simulink model "questao6"  (R2023a)
settings: Solver=VariableStepAuto  StartTime=0.0  StopTime=50  RelTol=1e-3
values from neighbouring files (symbols this model uses):
  B = 0.1    [Trab1_real.m]    (also in questao5.m)
  J = 1    [Trab1_real.m]    (also in questao5.m)
  K = 1/3    (= 0.333333333333)    [Trab1_real.m]    (also in questao5.m)
  L = 0.5    [Trab1_real.m]    (also in questao5.m)
  R = 10    [Trab1_real.m]    (also in questao5.m)
settings Model: Creator=thiag  LastModifiedBy=thiag

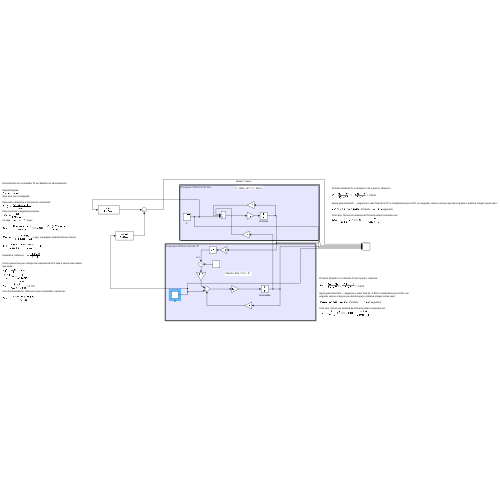
[thumbnail: Simulink's stored preview of the top-level diagram]
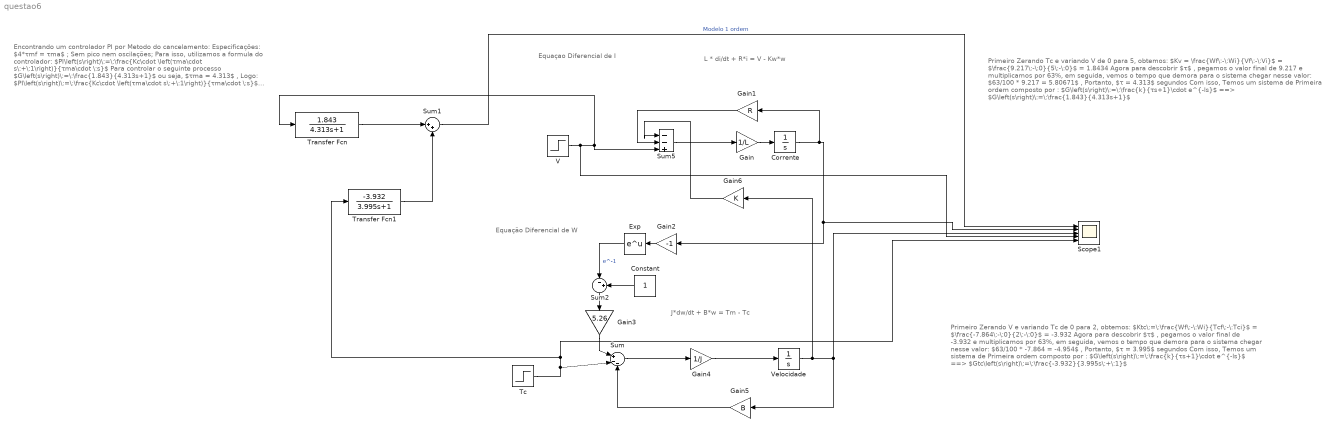
== system questao6 ==
  note: Encontrando um controlador PI por Metodo do cancelamento:
      |
      | Especificações:
      | $4*τmf = τma$ ;
      | Sem pico nem oscilações;
      |
      | Para isso, utilizamos a formula do controlador:
      | $PI\left(s\right)\:=\:\frac{Kc\cdot \left(τma\cdot s\:+\:1\right)}{τma\cdot \:s}$
      | Para controlar o seguinte processo
      | $G\left(s\right)\:=\:\frac{1.843}{4.313s+1}$
      | ou seja, $τma = 4.313$ , Logo:
      |
      | $PI\left(s\right)\:=\:\frac{Kc\cdot \left(τma\cdot s\:+\:1\right)}{τma\cdot \:s}$ ==> $PI\left(s\right)\:=\:\frac{Kc\cdot \left(4.313s+1\right)}{4.313s}$
      |
      | $Gmf\left(s\right)\:=\:\frac{C\left(s\right)\cdot G\left(s\right)}{1\:+\:C\left(s\right)\cdot G\left(S\right)}$ , Logo, a equação caracteristica se da por:
      |
      | $1\:+\:\frac{1.843}{4.313s+1}\cdot \frac{kc\left(4.313s+1\right)}{4.313s}\:=\:0$
      |
      | Isolando s, obtemos $s\:=\:\frac{-1.843kc}{4.313}$
      |
      | Como queremos que o tempo de resposta de Gmf seja 4 vezes mais rapido que Gma:
      | $τmf\:=\:\frac{τma}{4}\:\:=\:-\frac{1}{s}$
      | $\:\frac{4.313}{4}\:\:=\:-\frac{1}{\frac{-1.843Kc}{4.313}}$
      | $Kc\:\:=\frac{4\cdot 4.313}{\:4.313\:\cdot \:\:1.843}$ = 2.170
      | Com Kc Descoberto, obtemos nosso controlador, sendo ele:
      |
      | $PI\left(s\right)\:=\:\frac{2.170\:\cdot \:\left(4.313s+1\right)}{4.313s}$
  note: Primeiro Zerando V e variando Tc de 0 para 2, obtemos:
      |
      | $Ktc\:=\:\frac{Wf\:-\:Wi}{Tcf\:-\:Tci}$ = $\frac{-7.864\:-\:0}{2\:-\:0}$ = -3.932
      |
      | Agora para descobrir $τ$ , pegamos o valor final de -3.932 e multiplicamos por 63%, em seguida, vemos o tempo que demora para o sistema chegar nesse valor:
      |
      | $63/100 * -7.864 = -4.954$ , Portanto, $τ = 3.995$ segundos
      |
      | Com isso, Temos um sistema de Primeira ordem composto por :
      | $G\left(s\right)\:=\:\frac{k}{τs+1}\cdot e^{-ls}$ ==> $Gtc\left(s\right)\:=\:\frac{-3.932}{3.995s\:+\:1}$
  note: Primeiro Zerando Tc e variando V de 0 para 5, obtemos:
      |
      | $Kv = \frac{Wf\:-\:Wi}{Vf\:-\:Vi}$ = $\frac{9.217\:-\:0}{5\:-\:0}$ = 1.8434
      |
      | Agora para descobrir $τ$ , pegamos o valor final de 9.217 e multiplicamos por 63%, em seguida, vemos o tempo que demora para o sistema chegar nesse valor:
      |
      | $63/100 * 9.217 = 5.80671$ , Portanto, $τ = 4.313$ segundos
      |
      | Com isso, Temos um sistema de Primeira ordem composto por :
      | $G\left(s\right)\:=\:\frac{k}{τs+1}\cdot e^{-ls}$ ==> $G\left(s\right)\:=\:\frac{1.843}{4.313s+1}$
  note: J*dw/dt + B*w = Tm - Tc
  note: Equação Diferencial de W
  note: L * di/dt + R*i = V - Kw*w
  note: Equaçao Diferencial de I
  Constant : Constant
  Corrente : Integrator
  Exp : Math
  Gain : Gain  Gain=1/L
  Gain1 : Gain  Gain=R
  Gain2 : Gain  Gain=-1
  Gain3 : Gain  Gain=5.26
  Gain4 : Gain  Gain=1/J
  Gain5 : Gain  Gain=B
  Gain6 : Gain  Gain=K
  Scope1 : Scope  NumInputPorts=5
  Sum : Sum  Inputs=|+--
  Sum1 : Sum  Inputs=|++
  Sum2 : Sum  Inputs=|-+
  Sum5 : Sum  Inputs=|--+
  Tc : Step  Time=10  After=2  SampleTime=0
  Transfer Fcn : TransferFcn  Numerator=[1.843]  Denominator=[4.313 1]
  Transfer Fcn1 : TransferFcn  Numerator=[-3.932]  Denominator=[3.995 1]
  V : Step  Time=10  After=0  SampleTime=0
  Velocidade : Integrator
  wires:
  Velocidade/1 -> Scope1/3, Gain5/1, Gain6/1
  Gain/1 -> Corrente/1
  Gain3/1 -> Sum/1
  Gain2/1 -> Exp/1
  Constant/1 -> Sum2/2
  Gain5/1 -> Sum/3
  Sum2/1 -> Gain3/1
  Corrente/1 -> Gain2/1, Scope1/2, Gain1/1
  Exp/1 -> Sum2/1  "e^-1"
  Gain6/1 -> Sum5/1
  Gain4/1 -> Velocidade/1
  Gain1/1 -> Sum5/2
  Sum5/1 -> Gain/1
  Sum/1 -> Gain4/1
  V/1 -> Scope1/4, Transfer Fcn/1, Sum5/3
  Transfer Fcn/1 -> Sum1/1
  Transfer Fcn1/1 -> Sum1/2
  Tc/1 -> Transfer Fcn1/1, Scope1/5, Sum/2
  Sum1/1 -> Scope1/1  "Modelo 1 ordem"
